simulink model "penddemo"  (R2018a)
settings: Solver=ode45  StartTime=0  StopTime=10  MaxStep=0.02  RelTol=1e-3  AbsTol=1e-6
values from neighbouring files (symbols this model uses):
  A1 = A * dt + eye(4)    [penddemoExample.m]
  B1 = B * dt    [penddemoExample.m]
  C1 = eye(length(C))    [penddemoExample.m]
  C2 = [0 0 1 0]    [penddemoExample.m]
  D1 = zeros(size(B))    [penddemoExample.m]
undefined symbols (not defined in the file or in its folder): K
Description:
  | Inverted Pendulum with Animation
  | 
  | This example shows how to model an inverted pendulum.  The animation is created using MATLAB(R) Handle Graphics(R).  The animation block is a masked
  | S-function.  For more information, use the context menu to look under the Animation block's mask
  | and open the S-function for editing.
settings Model: ExtModeAutoUpdateStatusClock=off  Creator=The MathWorks, Inc.  LastModifiedBy=Brendon
settings SolverCC: AutoScaleAbsTol=off
settings DataIOCC: ExternalInput=[]  InitialState=[]  SaveFormat=Array  SaveOutput=off  SaveTime=off
settings OptimizationCC: BlockReduction=off  BooleanDataType=off  ExpressionDepthLimit=2147483647  InitFltsAndDblsToZero=on  LifeSpan=inf
settings DebuggingCC: SaveWithParameterizedLinksMsg=none  UnderspecifiedInitializationDetection=Classic  MergeDetectMultiDrivingBlocksExec=none  SignalResolutionControl=TryResolveAllWithWarning  MultiTaskDSMMsg=warning  MultiTaskCondExecSysMsg=none  SigSpecEnsureSampleTimeMsg=none  FcnCallInpInsideContextMsg=warning  StateNameClashWarn=warning  SFUnexpectedBacktrackingDiag=warning  SFNoUnconditionalDefaultTransitionDiag=warning  SFExecutionAtInitializationDiag=none
settings HardwareCC: ProdBitPerPointer=32  ProdBitPerSizeT=32  ProdBitPerPtrDiffT=32  ProdLargestAtomicFloat=None  ProdIntDivRoundTo=Undefined  ProdEndianess=Unspecified  ProdWordSize=32  ProdHWDeviceType=32-bit Generic  TargetUnknown=on
settings ModelReferenceCC: PropagateSignalLabelsOutOfModel=off
settings CodeAppCC: StateflowObjectComments=on
settings GRTTargetCC: TargetFcnLib=ansi_tfl_tmw.mat  TargetLangStandard=C89/C90 (ANSI)  GeneratePreprocessorConditionals=Disable all  CombineOutputUpdateFcns=off  GRTInterface=on
settings ConfigComp: CovMetricSettings=dw  CovHtmlReporting=on  CovSaveCumulativeToWorkspaceVar=on  CovSaveSingleToWorkspaceVar=on  CovExternalEMLEnable=off

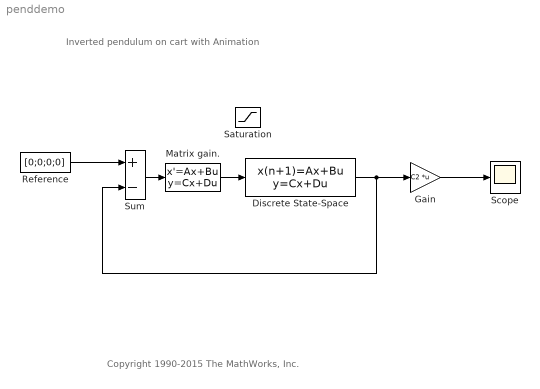
== system penddemo ==
  note: Inverted pendulum on cart with Animation
  note: Copyright 1990-2015 The MathWorks, Inc.
  Discrete State-Space : DiscreteStateSpace  A=A1  B=B1  C=C1  D=D1  InitialCondition=[0;0;0.1;0]  SampleTime=-1
  Gain : Gain  Gain=C2  Multiplication=Matrix(K*u)
  Matrix gain. : StateSpace  A=[]  B=[]  C=[]  D=K  InitialCondition=0  mask(Matrix gain){K=K}
      mask prompts: K "Gain matrix:"
      mask help: Matrix Gain:
      mask Help: Multiplies input vector by entered matrix to produce output vector.
      mask Display: disp('LQR')
  Reference : Constant  Value=[0;0;0;0]
  Saturation : Saturate  UpperLimit=10  LowerLimit=-10
  Scope : Scope
  Sum : Sum  Inputs=+-  SaturateOnIntegerOverflow=on  InputSameDT=on  OutDataTypeStr=Inherit: Same as first input
  wires:
  Discrete State-Space/1 -> Gain/1, Sum/2
  Reference/1 -> Sum/1
  Gain/1 -> Scope/1
  Sum/1 -> Matrix gain./1
  Matrix gain./1 -> Discrete State-Space/1
